simulink model "model"  (R2021b)
settings: Solver=VariableStepAuto  StartTime=0.0  StopTime=stop_czas  FixedStep=50  MaxStep=5  RelTol=1e-3
values from neighbouring files (symbols this model uses):
  cpow = 1000    [miniprojekt.m]
  Cvg = cpow*ppow*Vg    (= 1200)    [miniprojekt.m]
  Cvw = cpow*ppow*Vw    (= 36000)    [miniprojekt.m]
  dfg = 0    [miniprojekt.m]
  dqg = 0.1*qgN    (= 200)    [miniprojekt.m]
  dTzew = 1    [miniprojekt.m]
  fg = fgar(i)    [miniprojekt.m]
  K1 = (2*Kg*(TgN-TwewN))/(TwewN-TzewN)    (= 50)    [miniprojekt.m]
  Kg = qgN/(2*(TgN-TwewN))    (= 50)    [miniprojekt.m]
  ppow = 1.2    [miniprojekt.m]
  qg = qgar(i)    [miniprojekt.m]
  T = 1000    [miniprojekt.m]
  Tg0 = (qg*(Kg+K1+a)+(K1*Tzew)*(Kg+a))/((a+Kg)*(Kg+K1+a)-(a+Kg)^2)    [miniprojekt.m]
  Twew0 = (Tg0*(a+Kg)+K1*Tzew)/(Kg+K1+a)    [miniprojekt.m]
  Tzew = Tzewar(i)    [miniprojekt.m]
settings Model: Creator=jacek  LastModifiedBy=jacek

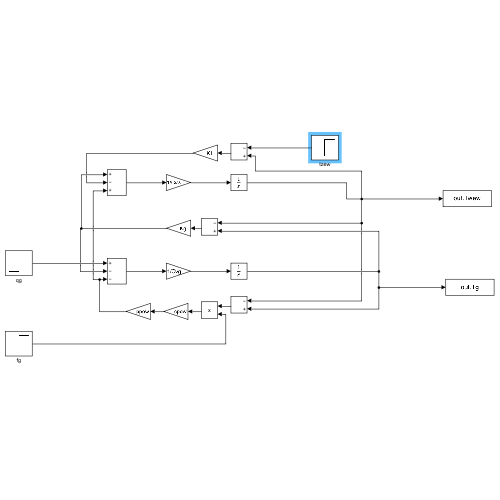
[thumbnail: Simulink's stored preview of the top-level diagram]
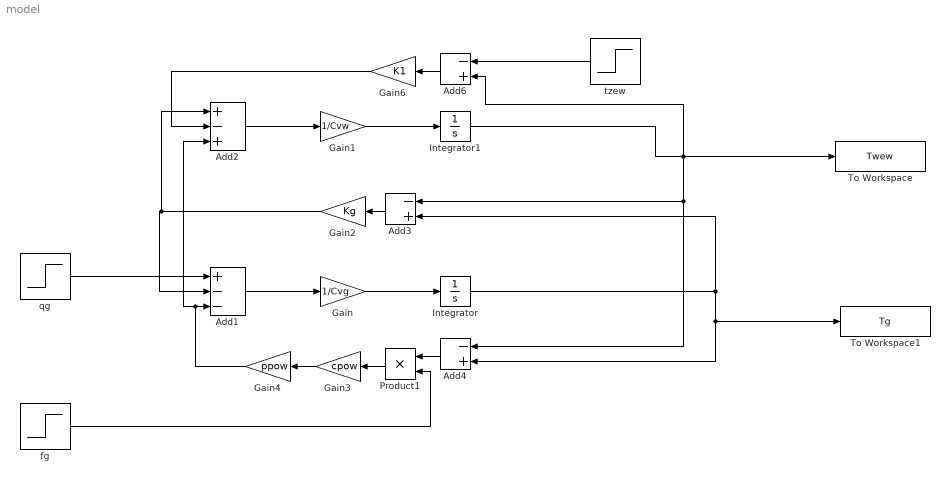
== system model ==
  Add1 : Sum  Inputs=+--
  Add2 : Sum  Inputs=+-+
  Add3 : Sum  Inputs=-+
  Add4 : Sum  Inputs=-+
  Add6 : Sum  Inputs=-+
  Gain : Gain  Gain=1/Cvg
  Gain1 : Gain  Gain=1/Cvw
  Gain2 : Gain  Gain=Kg
  Gain3 : Gain  Gain=cpow
  Gain4 : Gain  Gain=ppow
  Gain6 : Gain  Gain=K1
  Integrator : Integrator  InitialCondition=Tg0
  Integrator1 : Integrator  InitialCondition=Twew0
  Product1 : Product
  To Workspace : ToWorkspace  VariableName=Twew  SampleTime=-1
  To Workspace1 : ToWorkspace  VariableName=Tg  SampleTime=-1
  fg : Step  Time=T  Before=fg  After=dfg+fg  SampleTime=0
  qg : Step  Time=T  Before=qg  After=qg+dqg  SampleTime=0
  tzew : Step  Time=T  Before=Tzew  After=Tzew+dTzew  SampleTime=0
  wires:
  qg/1 -> Add1/1
  Gain/1 -> Integrator/1
  Add1/1 -> Gain/1
  Add2/1 -> Gain1/1
  Gain1/1 -> Integrator1/1
  Add3/1 -> Gain2/1
  Gain2/1 -> Add2/1, Add1/2
  Integrator1/1 -> Add3/1, Add4/1, Add6/2, To Workspace/1
  Integrator/1 -> Add4/2, To Workspace1/1, Add3/2
  fg/1 -> Product1/2
  Add4/1 -> Product1/1
  Product1/1 -> Gain3/1
  Gain3/1 -> Gain4/1
  Gain4/1 -> Add2/3, Add1/3
  Add6/1 -> Gain6/1
  tzew/1 -> Add6/1
  Gain6/1 -> Add2/2
